simulink model "furutaPend_fcn_sim"  (R2017b)
settings: Solver=ode4  StartTime=0.0  StopTime=10  FixedStep=0.001  RelTol=1e-3
libraries: vrlib x1
settings Model: Creator=ozhanyz  LastModifiedBy=ozhanyz
settings SolverCC: AlgebraicLoopSolver=LineSearch
settings DataIOCC: SaveFormat=Array

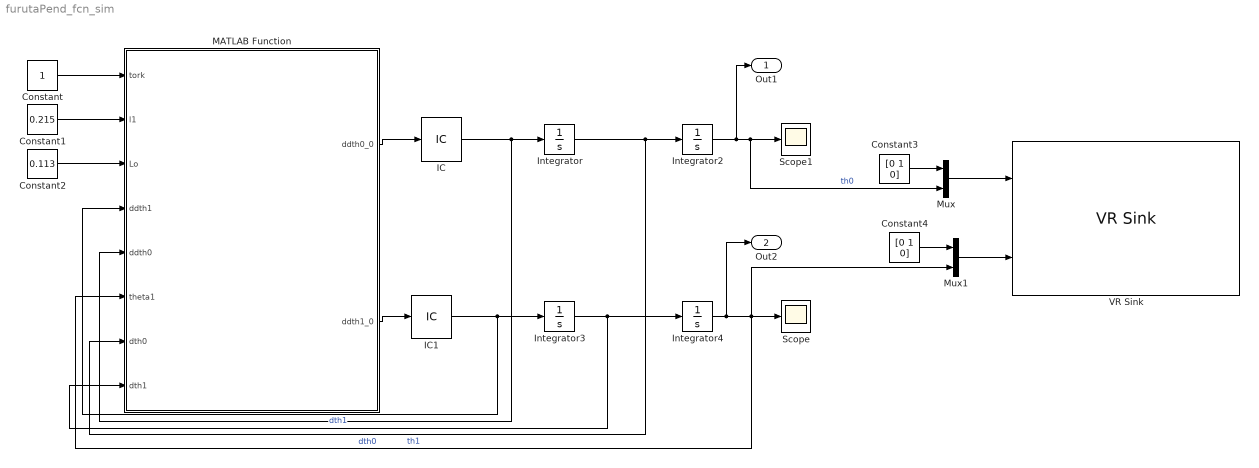
== system furutaPend_fcn_sim ==
  Constant : Constant
  Constant1 : Constant  Value=0.215
  Constant2 : Constant  Value=0.113
  Constant3 : Constant  Value=[0 1 0]
  Constant4 : Constant  Value=[0 1 0]
  IC : InitialCondition  Value=0.0000001
  IC1 : InitialCondition  Value=0.0000001
  Integrator{,2..4} (4 alike) : Integrator
  MATLAB Function : MATLAB Function  TreatAsAtomicUnit=on
  Mux : Mux  Inputs=2
  Mux1 : Mux  Inputs=2
  Scope : Scope
  Scope1 : Scope
  VR Sink : vrlib/VR Sink  InstantiateOnLoad=on  SampleTime=-1  ViewEnable=on  RemoteChange=off  RemoteView=off  FieldsWritten=Theta0.rotation.4.1.1.double#Theta1.rotation.4.1.1.double  WorldFileName=furutaPend_vrml.WRL  AutoView=off  VideoDimensions=[]  AllowVariableSize=off
      settings: SourceProductBaseCode=VR
  Out1 : Outport
  Out2 : Outport  Port=2
  wires:
  Integrator/1 -> MATLAB Function/7(dth0), Integrator2/1  "dth0"
  Integrator3/1 -> MATLAB Function/8(dth1), Integrator4/1  "dth1"
  MATLAB Function/2(ddth1_0) -> IC1/1
  Integrator4/1 -> Out2/1, Mux1/2, MATLAB Function/6(theta1), Scope/1  "th1"
  Integrator2/1 -> Out1/1, Mux/2, Scope1/1  "th0"
  MATLAB Function/1(ddth0_0) -> IC/1
  Constant/1 -> MATLAB Function/1(tork)
  IC/1 -> MATLAB Function/5(ddth0), Integrator/1
  IC1/1 -> MATLAB Function/4(ddth1), Integrator3/1
  Constant2/1 -> MATLAB Function/3(Lo)
  Constant1/1 -> MATLAB Function/2(l1)
  Constant4/1 -> Mux1/1
  Constant3/1 -> Mux/1
  Mux1/1 -> VR Sink/2
  Mux/1 -> VR Sink/1

== matlab function furutaPend_fcn_sim/MATLAB Function ==
  data: tork input; l1 input; Lo input; ddth0_0 output; ddth1 input; ddth0 input; theta1 input; dth0 input; dth1 input; ddth1_0 output
function[ddth0_0,ddth1_0] = furuta_Pend(tork,l1,Lo,ddth1,ddth0,theta1,dth0,dth1)
m=5.38*10^(-2);     Io=1.75*10^(-2);    
L1=0.25;            J1=1.98*10^(-4);
g=9.81;




ddth0_0=(tork-m*l1*(Lo*cos(theta1)*ddth1+l1*sin(2*theta1)*dth0*dth1-Lo*sin(theta1)*dth1*dth1))/(Io+m*Lo*Lo+l1*l1*m*sin(theta1)*sin(theta1));

ddth1_0=m*l1*(l1*sin(theta1)*cos(theta1)*(dth0^2)+g*sin(theta1)-Lo*cos(theta1)*dth0)/(J1+m*l1*l1);
